simulink model "control0"  (Simulink 8.1)
settings: Solver=ode45  StartTime=0.0  StopTime=10.0  RelTol=1e-3
values from neighbouring files (symbols this model uses):
  dc0 = [4]    [intro_sims.m]
  IC0 = 0.4/C0(2)    [intro_sims.m]
  nc0 = [3]    [intro_sims.m]
undefined symbols (not defined in the file or in its folder): A0, B0, C0, D0
libraries: simulink x2
settings Model: Creator=Dale  LastModifiedBy=MIZOPEX
settings DebuggingCC: StrictBusMsg=Warning

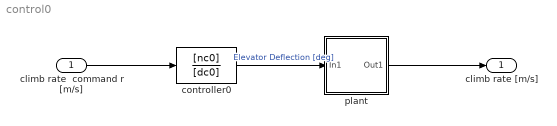
== system control0 ==
  climb rate  command r [m/s] : Inport
  controller0 : TransferFcn  Numerator=[nc0]  Denominator=[dc0]
  plant : Subsystem
  climb rate [m/s] : Outport
  wires:
  plant/1(Out1) -> climb rate [m/s]/1
  controller0/1 -> plant/1(In1)  "Elevator Deflection [deg]"
  climb rate  command r [m/s]/1 -> controller0/1

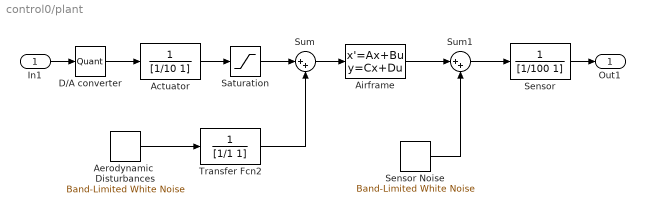
== system control0/plant ==
  In1 : Inport
  Actuator : TransferFcn  Denominator=[1/10 1]
  Aerodynamic  Disturbances : simulink/Sources/Band-Limited White Noise  Cov=[0.0]  Ts=0.01  seed=[13452]
  Airframe : StateSpace  A=A0  B=B0  C=C0  D=D0  X0=IC0
  D/A converter : Quantizer  QuantizationInterval=0.1
  Saturation : Saturate  UpperLimit=10  LowerLimit=-10
  Sensor : TransferFcn  Denominator=[1/100 1]
  Sensor Noise : simulink/Sources/Band-Limited White Noise  Cov=[0.00001]  Ts=0.01  seed=[23341]
  Sum : Sum  Inputs=|++
  Sum1 : Sum  Inputs=|++
  Transfer Fcn2 : TransferFcn  Denominator=[1/1 1]
  Out1 : Outport
  wires:
  D/A converter/1 -> Actuator/1
  Actuator/1 -> Saturation/1
  Saturation/1 -> Sum/1
  Sum/1 -> Airframe/1
  Airframe/1 -> Sum1/1
  Sum1/1 -> Sensor/1
  Aerodynamic  Disturbances/1 -> Transfer Fcn2/1
  Transfer Fcn2/1 -> Sum/2
  Sensor Noise/1 -> Sum1/2
  In1/1 -> D/A converter/1
  Sensor/1 -> Out1/1
